simulink model "mrefrobotarm_modified_previous_y_previous_u_previous_ref"  (R2018b)
settings: Solver=FixedStepAuto  StartTime=0.0  StopTime=10  RelTol=1e-3  AbsTol=1e-6
undefined symbols (not defined in the file or in its folder): options, sfunxy2
libraries: neural x949, simulink x1
(part 15 of 31)

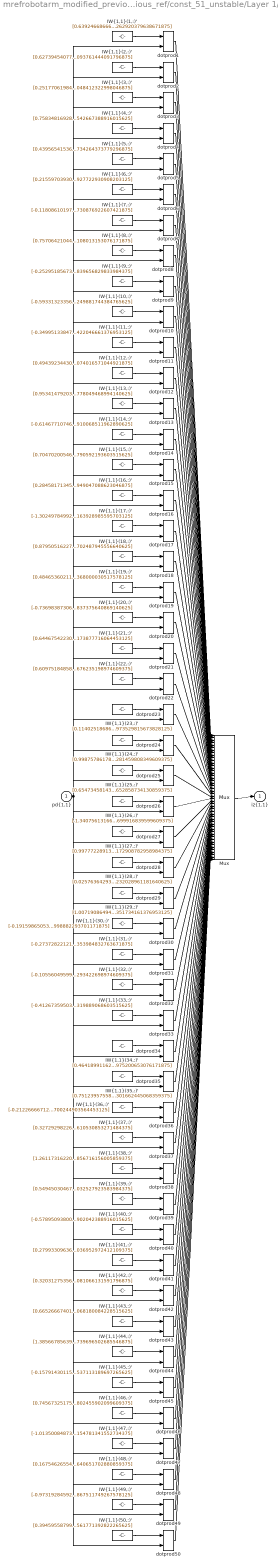
== system mrefrobotarm_modified_previous_y_previous_u_previous_ref/const_51_unstable/Layer 1/IW{1,1} ==
  "pd{1,1}" : Inport  PortDimensions=10
      mask Display: e = 0.06;c1 = [120 230 180]/255;c2 = ([120 230 180]+0)/(256+128);c3 = ([120 230 180]+128)/(256+128);patch([0 1 1 0],[0 0 1 1],c1);patch([0 1 1 1-e 1-e 0+e],[0 0 1 1-e 0+e 0+e],c2);patch([0 0 1 1-e 0+e 0+e],[0 1 1 1-e 1-e 0+e],c3);plot([0 1 1 0 0],[0 0 1 1 0]);
  "IW{1,1}(1,:)'" : Constant  Value=[0.63924668666616246692768754655844531953334808349609375;0.6942047904100672184313225443474948406219482421875;0.62567328865484228561655299927224405109882354736328125;0.261371173254488609050127934096963144838809967041015625;-0.177662377791001635518597367990878410637378692626953125;-0.8287859344063581712447330573922954499721527099609375;0.352973927789879848848642041048151440918445587158203125;0.2586532549009732395717264807899482548236846923828125;0.25408612949347031406688302013208158314228057861328125;-0.98861951008364001847183999416301958262920379638671875]
      mask Display: e = 0.06;c1 = [120 150 230]/255;c2 = ([120 150 230]+0)/383;c3 = ([120 150 230]+128)/383;patch([0 1 1 0],[0 0 1 1],c1);patch([0 1 1 1-e 1-e 0+e],[0 0 1 1-e 0+e 0+e],c2);patch([0 0 1 1-e 0+e 0+e],[0 1 1 1-e 1-e 0+e],c3);plot([0 1 1 0 0],[0 0 1 1 0]);disp('Weights');
  "IW{1,1}(10,:)'" : Constant  Value=[-0.59331323356992948792054676232510246336460113525390625;0.7977697325770243264031478247488848865032196044921875;-0.386101063294460644659267245515366084873676300048828125;-0.089448974061199615359640802125795744359493255615234375;0.50551080428874650696258186144405044615268707275390625;1.28460159328148382229528579046018421649932861328125;-1.051667369853578559713014328735880553722381591796875;-0.3071981244127155452616761976969428360462188720703125;-0.145228187797881769238728111304226331412792205810546875;0.416816636720638789004311774988309480249881744384765625]
      mask Display: e = 0.06;c1 = [120 150 230]/255;c2 = ([120 150 230]+0)/383;c3 = ([120 150 230]+128)/383;patch([0 1 1 0],[0 0 1 1],c1);patch([0 1 1 1-e 1-e 0+e],[0 0 1 1-e 0+e 0+e],c2);patch([0 0 1 1-e 0+e 0+e],[0 1 1 1-e 1-e 0+e],c3);plot([0 1 1 0 0],[0 0 1 1 0]);disp('Weights');
  "IW{1,1}(11,:)'" : Constant  Value=[-0.3499513384700432272467196526122279465198516845703125;-0.8005402749156467212543475397978909313678741455078125;-0.406764093260752357394949285662733018398284912109375;0.376972184217993555588321896721026860177516937255859375;-0.55931023341791130665257014697999693453311920166015625;-0.263639868612703442973810297189629636704921722412109375;-0.8852424690401410334317233719048090279102325439453125;0.51134822194627427283109000200056470930576324462890625;0.81875181176692046758347487411811016499996185302734375;0.45777739158591945756171526227262802422046661376953125]
      mask Display: e = 0.06;c1 = [120 150 230]/255;c2 = ([120 150 230]+0)/383;c3 = ([120 150 230]+128)/383;patch([0 1 1 0],[0 0 1 1],c1);patch([0 1 1 1-e 1-e 0+e],[0 0 1 1-e 0+e 0+e],c2);patch([0 0 1 1-e 0+e 0+e],[0 1 1 1-e 1-e 0+e],c3);plot([0 1 1 0 0],[0 0 1 1 0]);disp('Weights');
  "IW{1,1}(12,:)'" : Constant  Value=[0.494392344304093567242119888760498724877834320068359375;-1.09077574447859060313703594147227704524993896484375;-0.266408320699227540995224217112991027534008026123046875;-0.65079124667000576298647729345248080790042877197265625;-0.443937679832130116519550711018382571637630462646484375;0.334628474247073259828511027080821804702281951904296875;-0.7130336086197643918893618319998495280742645263671875;-1.161922006909116067419063256238587200641632080078125;-0.7882646426815498319484731837292201817035675048828125;-0.2961987538115529172699780247057788074016571044921875]
      mask Display: e = 0.06;c1 = [120 150 230]/255;c2 = ([120 150 230]+0)/383;c3 = ([120 150 230]+128)/383;patch([0 1 1 0],[0 0 1 1],c1);patch([0 1 1 1-e 1-e 0+e],[0 0 1 1-e 0+e 0+e],c2);patch([0 0 1 1-e 0+e 0+e],[0 1 1 1-e 1-e 0+e],c3);plot([0 1 1 0 0],[0 0 1 1 0]);disp('Weights');
  "IW{1,1}(13,:)'" : Constant  Value=[0.95341479203810586273704075210844166576862335205078125;-0.8400060597329204181704653819906525313854217529296875;-0.7955112231704415393096496700309216976165771484375;0.9668516464493592810214295241166837513446807861328125;-0.59452250697652286870464877210906706750392913818359375;-0.8387872006048218143092753962264396250247955322265625;0.15730537243195630292547093631583265960216522216796875;0.01305569298102214094436934743725942098535597324371337890625;-0.0997248402186528271062826433990267105400562286376953125;-0.048607066451850290678127208821024396456778049468994140625]
      mask Display: e = 0.06;c1 = [120 150 230]/255;c2 = ([120 150 230]+0)/383;c3 = ([120 150 230]+128)/383;patch([0 1 1 0],[0 0 1 1],c1);patch([0 1 1 1-e 1-e 0+e],[0 0 1 1-e 0+e 0+e],c2);patch([0 0 1 1-e 0+e 0+e],[0 1 1 1-e 1-e 0+e],c3);plot([0 1 1 0 0],[0 0 1 1 0]);disp('Weights');
  "IW{1,1}(14,:)'" : Constant  Value=[-0.61467710746125892029567694407887756824493408203125;-0.74682779167762614047632041547331027686595916748046875;-0.473858474488004943747654351682285778224468231201171875;-0.95402929876217867910526138075510971248149871826171875;0.333174273926396036227259855877491645514965057373046875;-0.36303307199912338010250323350192047655582427978515625;0.81652223062918627416451045064604841172695159912109375;0.2424313956082983778639317051784018985927104949951171875;-0.79565150315721100415800037808367051184177398681640625;-0.5094853025869279239401521408581174910068511962890625]
      mask Display: e = 0.06;c1 = [120 150 230]/255;c2 = ([120 150 230]+0)/383;c3 = ([120 150 230]+128)/383;patch([0 1 1 0],[0 0 1 1],c1);patch([0 1 1 1-e 1-e 0+e],[0 0 1 1-e 0+e 0+e],c2);patch([0 0 1 1-e 0+e 0+e],[0 1 1 1-e 1-e 0+e],c3);plot([0 1 1 0 0],[0 0 1 1 0]);disp('Weights');
  "IW{1,1}(15,:)'" : Constant  Value=[0.70470200546815409126111262594349682331085205078125;0.9721504333185293500463330929051153361797332763671875;0.626300057389828079834614982246421277523040771484375;0.213189582099907293244456241154693998396396636962890625;0.6913359965783083538326536654494702816009521484375;-0.00295197046113919621401766590906845522113144397735595703125;-0.8625857589857603979766054180799983441829681396484375;0.59018061405102095751118440603022463619709014892578125;0.90924827447133338420570680682430975139141082763671875;0.85333254725311835642287405789829790592193603515625]
      mask Display: e = 0.06;c1 = [120 150 230]/255;c2 = ([120 150 230]+0)/383;c3 = ([120 150 230]+128)/383;patch([0 1 1 0],[0 0 1 1],c1);patch([0 1 1 1-e 1-e 0+e],[0 0 1 1-e 0+e 0+e],c2);patch([0 0 1 1-e 0+e 0+e],[0 1 1 1-e 1-e 0+e],c3);plot([0 1 1 0 0],[0 0 1 1 0]);disp('Weights');
  "IW{1,1}(16,:)'" : Constant  Value=[0.284581713458217089307566993738873861730098724365234375;-0.280621549126129188334033415230805985629558563232421875;-1.03564915596999451707915795850567519664764404296875;-0.07172317120460820760730058509579976089298725128173828125;0.39460759001793388467405065966886468231678009033203125;0.9190004709601919952177695449790917336940765380859375;0.75048181864749563541039378833374939858913421630859375;0.81573633636398434898495679590268991887569427490234375;-0.03591301039200699152242890477282344363629817962646484375;0.85062050036111880313427491273614577949047088623046875]
      mask Display: e = 0.06;c1 = [120 150 230]/255;c2 = ([120 150 230]+0)/383;c3 = ([120 150 230]+128)/383;patch([0 1 1 0],[0 0 1 1],c1);patch([0 1 1 1-e 1-e 0+e],[0 0 1 1-e 0+e 0+e],c2);patch([0 0 1 1-e 0+e 0+e],[0 1 1 1-e 1-e 0+e],c3);plot([0 1 1 0 0],[0 0 1 1 0]);disp('Weights');
  "IW{1,1}(17,:)'" : Constant  Value=[-1.3024978499248760499540367163717746734619140625;1.3419509605779460503782729574595578014850616455078125;-0.504540389310853765181263952399604022502899169921875;0.5007126364069047763649678017827682197093963623046875;-0.2241232702447646107923873159961658529937267303466796875;-0.682842349014617155944506521336734294891357421875;-0.59445267552896596807698870179592631757259368896484375;1.2325888373718640877996222116053104400634765625;-0.0831161952569162976178773760693729855120182037353515625;-0.565871713313782720433664508163928985595703125]
      mask Display: e = 0.06;c1 = [120 150 230]/255;c2 = ([120 150 230]+0)/383;c3 = ([120 150 230]+128)/383;patch([0 1 1 0],[0 0 1 1],c1);patch([0 1 1 1-e 1-e 0+e],[0 0 1 1-e 0+e 0+e],c2);patch([0 0 1 1-e 0+e 0+e],[0 1 1 1-e 1-e 0+e],c3);plot([0 1 1 0 0],[0 0 1 1 0]);disp('Weights');
  "IW{1,1}(18,:)'" : Constant  Value=[0.87950516227352704135000749374739825725555419921875;-1.1836890447335763898450977649190463125705718994140625;0.530743319631852283890793842147104442119598388671875;0.25272269822145509987620926040108315646648406982421875;0.3653029490932790945834085505339317023754119873046875;-0.3810355298209933128106285948888398706912994384765625;-0.64649896901114478620087311355746351182460784912109375;0.300211636084151523018448415314196608960628509521484375;-0.428387989166555904763100670606945641338825225830078125;0.1751370188022575435926597720026620663702487945556640625]
      mask Display: e = 0.06;c1 = [120 150 230]/255;c2 = ([120 150 230]+0)/383;c3 = ([120 150 230]+128)/383;patch([0 1 1 0],[0 0 1 1],c1);patch([0 1 1 1-e 1-e 0+e],[0 0 1 1-e 0+e 0+e],c2);patch([0 0 1 1-e 0+e 0+e],[0 1 1 1-e 1-e 0+e],c3);plot([0 1 1 0 0],[0 0 1 1 0]);disp('Weights');
  "IW{1,1}(19,:)'" : Constant  Value=[0.48465360211071384366476877403329126536846160888671875;-0.71564584780320006363041329677798785269260406494140625;-0.1134074702547006319175437738522305153310298919677734375;-0.38993116043481312882335032554692588746547698974609375;-0.6878127659446697794720648744259960949420928955078125;0.364118141393751260093125665662228129804134368896484375;0.472555272999996500704611435139668174088001251220703125;0.1810251256197520641766374183134757913649082183837890625;-0.86523040981986676367654354180558584630489349365234375;0.479601809228045461441780616951291449368000030517578125]
      mask Display: e = 0.06;c1 = [120 150 230]/255;c2 = ([120 150 230]+0)/383;c3 = ([120 150 230]+128)/383;patch([0 1 1 0],[0 0 1 1],c1);patch([0 1 1 1-e 1-e 0+e],[0 0 1 1-e 0+e 0+e],c2);patch([0 0 1 1-e 0+e 0+e],[0 1 1 1-e 1-e 0+e],c3);plot([0 1 1 0 0],[0 0 1 1 0]);disp('Weights');
  "IW{1,1}(2,:)'" : Constant  Value=[0.62739454077566769729656925846938975155353546142578125;0.76646187434358548085100437674554996192455291748046875;0.8709533037536247856991167282103560864925384521484375;-0.7335425158669657275112285788054578006267547607421875;-0.2353430122977316074628362230214406736195087432861328125;0.81640575167049933558161001201369799673557281494140625;0.72409700386967756902123483087052591145038604736328125;0.45266443098558573066014787400490604341030120849609375;0.1720296099524863675522823314167908392846584320068359375;-1.033946502245487675253343695658259093761444091796875]
      mask Display: e = 0.06;c1 = [120 150 230]/255;c2 = ([120 150 230]+0)/383;c3 = ([120 150 230]+128)/383;patch([0 1 1 0],[0 0 1 1],c1);patch([0 1 1 1-e 1-e 0+e],[0 0 1 1-e 0+e 0+e],c2);patch([0 0 1 1-e 0+e 0+e],[0 1 1 1-e 1-e 0+e],c3);plot([0 1 1 0 0],[0 0 1 1 0]);disp('Weights');
  "IW{1,1}(20,:)'" : Constant  Value=[-0.7369838730691868899924656943767331540584564208984375;-0.45128021209423885284905963999335654079914093017578125;0.84230940906155671310528987305588088929653167724609375;-0.13210537730959004409925228173960931599140167236328125;-0.0816075728062311822608165812198421917855739593505859375;-0.022981247943674322498086581845200271345674991607666015625;-0.41000811331266484582869225050671957433223724365234375;-0.77313035067709401371160993221565149724483489990234375;1.1472657437635669364084378685220144689083099365234375;0.65177088639075508869069608408608473837375640869140625]
      mask Display: e = 0.06;c1 = [120 150 230]/255;c2 = ([120 150 230]+0)/383;c3 = ([120 150 230]+128)/383;patch([0 1 1 0],[0 0 1 1],c1);patch([0 1 1 1-e 1-e 0+e],[0 0 1 1-e 0+e 0+e],c2);patch([0 0 1 1-e 0+e 0+e],[0 1 1 1-e 1-e 0+e],c3);plot([0 1 1 0 0],[0 0 1 1 0]);disp('Weights');
  "IW{1,1}(21,:)'" : Constant  Value=[0.64467542230901309086021910843555815517902374267578125;-0.365686964333162556339829052376444451510906219482421875;-1.1167429230065206713362613299977965652942657470703125;-0.28027872976577128394382043552468530833721160888671875;-1.15425342475938119690681560314260423183441162109375;0.00147963811568855956035672960524607333354651927947998046875;-0.58953701284011483796376751342904753983020782470703125;-0.8196672851852664365424061543308198451995849609375;0.5859115741298446256024590184097178280353546142578125;-0.232936107706306405606966336563345976173877716064453125]
      mask Display: e = 0.06;c1 = [120 150 230]/255;c2 = ([120 150 230]+0)/383;c3 = ([120 150 230]+128)/383;patch([0 1 1 0],[0 0 1 1],c1);patch([0 1 1 1-e 1-e 0+e],[0 0 1 1-e 0+e 0+e],c2);patch([0 0 1 1-e 0+e 0+e],[0 1 1 1-e 1-e 0+e],c3);plot([0 1 1 0 0],[0 0 1 1 0]);disp('Weights');
  "IW{1,1}(22,:)'" : Constant  Value=[0.60975184858876441129638124039047397673130035400390625;-1.1137511038478298264209342960384674370288848876953125;0.75737428038547705000382848083972930908203125;-0.949374181419179397067864556447602808475494384765625;-0.05697986041225151787603664388370816595852375030517578125;-0.232736767374490505222439651333843357861042022705078125;-0.306641934219895606617001249105669558048248291015625;0.5422382160818004503965994445024989545345306396484375;0.355223820942887125173825779711478389799594879150390625;0.520671647549169502866561742848716676235198974609375]
      mask Display: e = 0.06;c1 = [120 150 230]/255;c2 = ([120 150 230]+0)/383;c3 = ([120 150 230]+128)/383;patch([0 1 1 0],[0 0 1 1],c1);patch([0 1 1 1-e 1-e 0+e],[0 0 1 1-e 0+e 0+e],c2);patch([0 0 1 1-e 0+e 0+e],[0 1 1 1-e 1-e 0+e],c3);plot([0 1 1 0 0],[0 0 1 1 0]);disp('Weights');
  "IW{1,1}(23,:)'" : Constant  Value=[0.11402518686013463078410268281004391610622406005859375;0.4904421195008132894344043961609713733196258544921875;0.68664774896037561457973197320825420320034027099609375;0.51860306312847981313751688503543846309185028076171875;-0.6427156453918172474004677496850490570068359375;-0.9590374190953838695605782049824483692646026611328125;0.0373927440447821834990094203021726571023464202880859375;0.68495669364243438881345582558424212038516998291015625;0.94546553725292736825025485813966952264308929443359375;-0.339602270344673329294238328657229430973529815673828125]
      mask Display: e = 0.06;c1 = [120 150 230]/255;c2 = ([120 150 230]+0)/383;c3 = ([120 150 230]+128)/383;patch([0 1 1 0],[0 0 1 1],c1);patch([0 1 1 1-e 1-e 0+e],[0 0 1 1-e 0+e 0+e],c2);patch([0 0 1 1-e 0+e 0+e],[0 1 1 1-e 1-e 0+e],c3);plot([0 1 1 0 0],[0 0 1 1 0]);disp('Weights');
  "IW{1,1}(24,:)'" : Constant  Value=[0.9987578617813903658628760240389965474605560302734375;0.495486441201053506855345176518312655389308929443359375;-0.2127739742921361532079771450298721902072429656982421875;0.8271982061539644437431206824840046465396881103515625;-0.410956095251641340126980139757506549358367919921875;-0.7970129128845797605862344425986520946025848388671875;0.9105423389600943995247916973312385380268096923828125;0.90778107591924384056625285666086710989475250244140625;-0.506466458102025729459683134336955845355987548828125;0.354856883470640871447443487340933643281459808349609375]
      mask Display: e = 0.06;c1 = [120 150 230]/255;c2 = ([120 150 230]+0)/383;c3 = ([120 150 230]+128)/383;patch([0 1 1 0],[0 0 1 1],c1);patch([0 1 1 1-e 1-e 0+e],[0 0 1 1-e 0+e 0+e],c2);patch([0 0 1 1-e 0+e 0+e],[0 1 1 1-e 1-e 0+e],c3);plot([0 1 1 0 0],[0 0 1 1 0]);disp('Weights');
  "IW{1,1}(25,:)'" : Constant  Value=[0.6547345814357929949522940660244785249233245849609375;0.39845260412756022816438417066819965839385986328125;-0.1830170343104607078021928145972196944057941436767578125;1.3632995620440577777543467163923196494579315185546875;0.80754118590340340233524329960346221923828125;0.381451563537807292192383101792074739933013916015625;0.71053106300381696502910244817030616104602813720703125;-0.63610894017396069077818765435949899256229400634765625;0.363044771167251700827449667485780082643032073974609375;-0.042781005916550096657147150835953652858734130859375]
      mask Display: e = 0.06;c1 = [120 150 230]/255;c2 = ([120 150 230]+0)/383;c3 = ([120 150 230]+128)/383;patch([0 1 1 0],[0 0 1 1],c1);patch([0 1 1 1-e 1-e 0+e],[0 0 1 1-e 0+e 0+e],c2);patch([0 0 1 1-e 0+e 0+e],[0 1 1 1-e 1-e 0+e],c3);plot([0 1 1 0 0],[0 0 1 1 0]);disp('Weights');
  "IW{1,1}(26,:)'" : Constant  Value=[-1.340756131664672334835586298140697181224822998046875;0.27007456478198499372211927038733847439289093017578125;-0.039195464485621826777883569548066589049994945526123046875;-0.62996699208041062600926807135692797601222991943359375;1.24456451050825744886196844163350760936737060546875;-0.25402186930486736482492915456532500684261322021484375;0.29241835179487962736999406843096949160099029541015625;-0.2364904402252494819425265859536011703312397003173828125;-0.56760479989431023017942834485438652336597442626953125;0.419969212660492308142323736319667659699916839599609375]
      mask Display: e = 0.06;c1 = [120 150 230]/255;c2 = ([120 150 230]+0)/383;c3 = ([120 150 230]+128)/383;patch([0 1 1 0],[0 0 1 1],c1);patch([0 1 1 1-e 1-e 0+e],[0 0 1 1-e 0+e 0+e],c2);patch([0 0 1 1-e 0+e 0+e],[0 1 1 1-e 1-e 0+e],c3);plot([0 1 1 0 0],[0 0 1 1 0]);disp('Weights');
  "IW{1,1}(27,:)'" : Constant  Value=[0.9977722891376490377268737574922852218151092529296875;-0.6068679135028485216452054373803548514842987060546875;0.50421216035368698893393002435914240777492523193359375;0.311630050128098357031802834171685390174388885498046875;-0.37280063608242486328236964254756458103656768798828125;0.97080864432455837853552793603739701211452484130859375;-1.060044686277588521505776952835731208324432373046875;0.97769244225342089027463998718303628265857696533203125;-0.329571569628752059077925196106662042438983917236328125;-0.456574952393950128648469899417250417172908782958984375]
      mask Display: e = 0.06;c1 = [120 150 230]/255;c2 = ([120 150 230]+0)/383;c3 = ([120 150 230]+128)/383;patch([0 1 1 0],[0 0 1 1],c1);patch([0 1 1 1-e 1-e 0+e],[0 0 1 1-e 0+e 0+e],c2);patch([0 0 1 1-e 0+e 0+e],[0 1 1 1-e 1-e 0+e],c3);plot([0 1 1 0 0],[0 0 1 1 0]);disp('Weights');
  "IW{1,1}(28,:)'" : Constant  Value=[0.02576364293666101590307704327642568387091159820556640625;-0.65255059643876556219055373730952851474285125732421875;-0.87832867100243394720138212505844421684741973876953125;-0.778813682076582747271231710328720510005950927734375;-0.709411760323691797935907743521966040134429931640625;0.5312754913211226170943746183183975517749786376953125;0.501196663942328424212746540433727204799652099609375;-0.6671465678213934769047455120016820728778839111328125;-0.56260016957891745281727935434901155531406402587890625;-0.56810980620226703141639745808788575232028961181640625]
      mask Display: e = 0.06;c1 = [120 150 230]/255;c2 = ([120 150 230]+0)/383;c3 = ([120 150 230]+128)/383;patch([0 1 1 0],[0 0 1 1],c1);patch([0 1 1 1-e 1-e 0+e],[0 0 1 1-e 0+e 0+e],c2);patch([0 0 1 1-e 0+e 0+e],[0 1 1 1-e 1-e 0+e],c3);plot([0 1 1 0 0],[0 0 1 1 0]);disp('Weights');
  "IW{1,1}(29,:)'" : Constant  Value=[1.0071908649480600939085661593708209693431854248046875;-0.59269777759990216470242785362643189728260040283203125;0.6430474184332164444555246518575586378574371337890625;-0.177195096398686136041078498237766325473785400390625;0.64647725132764144451158472293172962963581085205078125;-1.0737955968979908671911971396184526383876800537109375;0.32481199487106326984076076769270002841949462890625;0.2653582624213639551413734807283617556095123291015625;0.32551897435131615932135673574521206319332122802734375;0.421670984283849581419900687251356430351734161376953125]
      mask Display: e = 0.06;c1 = [120 150 230]/255;c2 = ([120 150 230]+0)/383;c3 = ([120 150 230]+128)/383;patch([0 1 1 0],[0 0 1 1],c1);patch([0 1 1 1-e 1-e 0+e],[0 0 1 1-e 0+e 0+e],c2);patch([0 0 1 1-e 0+e 0+e],[0 1 1 1-e 1-e 0+e],c3);plot([0 1 1 0 0],[0 0 1 1 0]);disp('Weights');
  "IW{1,1}(3,:)'" : Constant  Value=[0.251770619842439924429555730966967530548572540283203125;-0.29186179488348640287398438886157236993312835693359375;0.2317864436403720418411467107944190502166748046875;0.346406667185564176580925277448841370642185211181640625;-1.1818576323231848590467052417807281017303466796875;0.6938375834008052578383285435847938060760498046875;-0.95315078904075634103065794988651759922504425048828125;0.036065412262522460185021344614142435602843761444091796875;-0.6930875611524214274794530865619890391826629638671875;-0.72257924625952252295491007316741161048412322998046875]
      mask Display: e = 0.06;c1 = [120 150 230]/255;c2 = ([120 150 230]+0)/383;c3 = ([120 150 230]+128)/383;patch([0 1 1 0],[0 0 1 1],c1);patch([0 1 1 1-e 1-e 0+e],[0 0 1 1-e 0+e 0+e],c2);patch([0 0 1 1-e 0+e 0+e],[0 1 1 1-e 1-e 0+e],c3);plot([0 1 1 0 0],[0 0 1 1 0]);disp('Weights');
  "IW{1,1}(30,:)'" : Constant  Value=[-0.19159865053693125869216373757808469235897064208984375;-1.044827388502894915944807507912628352642059326171875;-0.95362540357193303908189818685059435665607452392578125;0.9439417571944748175383210764266550540924072265625;-0.776251292475051979380396005581133067607879638671875;0.062431350981061985161435501368032419122755527496337890625;-0.07510985747671532208880051939559052698314189910888671875;0.2325848996406161550698499240752425976097583770751953125;-0.441251057412189340301011952760745771229267120361328125;-0.1266650210668011922177100814224104396998882293701171875]
      mask Display: e = 0.06;c1 = [120 150 230]/255;c2 = ([120 150 230]+0)/383;c3 = ([120 150 230]+128)/383;patch([0 1 1 0],[0 0 1 1],c1);patch([0 1 1 1-e 1-e 0+e],[0 0 1 1-e 0+e 0+e],c2);patch([0 0 1 1-e 0+e 0+e],[0 1 1 1-e 1-e 0+e],c3);plot([0 1 1 0 0],[0 0 1 1 0]);disp('Weights');
  "IW{1,1}(31,:)'" : Constant  Value=[-0.27372822121770479242286455701105296611785888671875;-0.216348771194250166782779842833406291902065277099609375;-0.72304138575442433722884061353397555649280548095703125;-0.64024653526934127700798171645146794617176055908203125;-0.54564834135397799474986868517589755356311798095703125;1.00143652126254867340549026266671717166900634765625;-0.65234906555163518770967812088201753795146942138671875;-0.69565204535261149221270216003176756203174591064453125;-0.422829370206151355926493806691723875701427459716796875;0.79132190290408288557699734155903570353984832763671875]
      mask Display: e = 0.06;c1 = [120 150 230]/255;c2 = ([120 150 230]+0)/383;c3 = ([120 150 230]+128)/383;patch([0 1 1 0],[0 0 1 1],c1);patch([0 1 1 1-e 1-e 0+e],[0 0 1 1-e 0+e 0+e],c2);patch([0 0 1 1-e 0+e 0+e],[0 1 1 1-e 1-e 0+e],c3);plot([0 1 1 0 0],[0 0 1 1 0]);disp('Weights');
  "IW{1,1}(32,:)'" : Constant  Value=[-0.10556049599311063957873813023979892022907733917236328125;0.00584291461163955437585482144413617788814008235931396484375;-1.3863775039244092823764731292612850666046142578125;-0.2103211703886511685368532198481261730194091796875;-1.2577814118814940602675278569222427904605865478515625;0.05686350527750520800207567617690074257552623748779296875;0.40230834706792129029651050586835481226444244384765625;0.345830932655557699018089579112711362540721893310546875;-0.058080826938076889065509789134011953137814998626708984375;-0.78958512148689441456639315219945274293422698974609375]
      mask Display: e = 0.06;c1 = [120 150 230]/255;c2 = ([120 150 230]+0)/383;c3 = ([120 150 230]+128)/383;patch([0 1 1 0],[0 0 1 1],c1);patch([0 1 1 1-e 1-e 0+e],[0 0 1 1-e 0+e 0+e],c2);patch([0 0 1 1-e 0+e 0+e],[0 1 1 1-e 1-e 0+e],c3);plot([0 1 1 0 0],[0 0 1 1 0]);disp('Weights');
  "IW{1,1}(33,:)'" : Constant  Value=[-0.412673595033445028690266553894616663455963134765625;-0.61251027096036037011828057075035758316516876220703125;0.31789585632212757904113686890923418104648590087890625;0.49313760996205580067197615790064446628093719482421875;-0.76689035985725428901105260592885315418243408203125;0.92766504905938484970562285525375045835971832275390625;-0.81904960000742443870791476001613773405551910400390625;0.418870210355308192351486695770290680229663848876953125;0.0958785722800684914179925044663832522928714752197265625;0.393281295541891451339466811987222172319889068603515625]
      mask Display: e = 0.06;c1 = [120 150 230]/255;c2 = ([120 150 230]+0)/383;c3 = ([120 150 230]+128)/383;patch([0 1 1 0],[0 0 1 1],c1);patch([0 1 1 1-e 1-e 0+e],[0 0 1 1-e 0+e 0+e],c2);patch([0 0 1 1-e 0+e 0+e],[0 1 1 1-e 1-e 0+e],c3);plot([0 1 1 0 0],[0 0 1 1 0]);disp('Weights');
  "IW{1,1}(34,:)'" : Constant  Value=[0.4641899116284331494597381606581620872020721435546875;1.058282155187232564941268719849176704883575439453125;-0.302014535432015396310134747182019054889678955078125;-0.6903925305826994485158820680226199328899383544921875;0.61960402696297156577287523759878240525722503662109375;0.82478305479356517349032174024614505469799041748046875;-0.57352396235207991903592983362614177167415618896484375;0.1844165746886447243557682895698235370218753814697265625;1.063607222221527148775521709467284381389617919921875;0.030075523509437478153483169762694160453975200653076171875]
      mask Display: e = 0.06;c1 = [120 150 230]/255;c2 = ([120 150 230]+0)/383;c3 = ([120 150 230]+128)/383;patch([0 1 1 0],[0 0 1 1],c1);patch([0 1 1 1-e 1-e 0+e],[0 0 1 1-e 0+e 0+e],c2);patch([0 0 1 1-e 0+e 0+e],[0 1 1 1-e 1-e 0+e],c3);plot([0 1 1 0 0],[0 0 1 1 0]);disp('Weights');
  "IW{1,1}(35,:)'" : Constant  Value=[0.75123957558842124893061509283143095672130584716796875;-0.7965275034147210053703247467637993395328521728515625;0.045205342260291096756485984542450751177966594696044921875;-0.5146427157032678056935992572107352316379547119140625;-1.170604211533416094681570029933936893939971923828125;1.1039268224372966731294809505925513803958892822265625;-0.437798827711881555213579986229888163506984710693359375;0.336384367120219851532425536788650788366794586181640625;0.1421463715218020673614063298373366706073284149169921875;0.73457620854121896680766212739399634301662445068359375]
      mask Display: e = 0.06;c1 = [120 150 230]/255;c2 = ([120 150 230]+0)/383;c3 = ([120 150 230]+128)/383;patch([0 1 1 0],[0 0 1 1],c1);patch([0 1 1 1-e 1-e 0+e],[0 0 1 1-e 0+e 0+e],c2);patch([0 0 1 1-e 0+e 0+e],[0 1 1 1-e 1-e 0+e],c3);plot([0 1 1 0 0],[0 0 1 1 0]);disp('Weights');
  "IW{1,1}(36,:)'" : Constant  Value=[-0.2122666671298679974544398874058970250189304351806640625;0.76651151168379116906947956522344611585140228271484375;-0.0003967882681511071367441711998935716110281646251678466796875;0.44828287097590535648095055876183323562145233154296875;-0.5292928794968714267810128148994408547878265380859375;-0.8290689229590098019428978659561835229396820068359375;0.348926523801390942036704245765577070415019989013671875;1.014816697147457258409986025071702897548675537109375;-1.11439146435958935654753076960332691669464111328125;0.314956379104058659113007934138295240700244903564453125]
      mask Display: e = 0.06;c1 = [120 150 230]/255;c2 = ([120 150 230]+0)/383;c3 = ([120 150 230]+128)/383;patch([0 1 1 0],[0 0 1 1],c1);patch([0 1 1 1-e 1-e 0+e],[0 0 1 1-e 0+e 0+e],c2);patch([0 0 1 1-e 0+e 0+e],[0 1 1 1-e 1-e 0+e],c3);plot([0 1 1 0 0],[0 0 1 1 0]);disp('Weights');
  "IW{1,1}(37,:)'" : Constant  Value=[0.327292982263773513107452117765205912292003631591796875;0.8200236668707205911488244964857585728168487548828125;-0.201589082457516166613231689552776515483856201171875;0.37970567032044943989177454568562097847461700439453125;-0.61236992485544139430686527703073807060718536376953125;0.6132460084698820867998847461421974003314971923828125;-0.054611185509608493882094393256920739077031612396240234375;0.1957005208180704614040479327741195447742938995361328125;1.1601839643593023776446671035955660045146942138671875;-0.66306043780564338785410427590250037610530853271484375]
      mask Display: e = 0.06;c1 = [120 150 230]/255;c2 = ([120 150 230]+0)/383;c3 = ([120 150 230]+128)/383;patch([0 1 1 0],[0 0 1 1],c1);patch([0 1 1 1-e 1-e 0+e],[0 0 1 1-e 0+e 0+e],c2);patch([0 0 1 1-e 0+e 0+e],[0 1 1 1-e 1-e 0+e],c3);plot([0 1 1 0 0],[0 0 1 1 0]);disp('Weights');
  "IW{1,1}(38,:)'" : Constant  Value=[1.2611731622048385492718125533428974449634552001953125;0.75217689002794940744678342525730840861797332763671875;-0.44177672716117732942819884556229226291179656982421875;0.1614755608187066482361871067041647620499134063720703125;0.56127082889771517937305134182679466903209686279296875;0.06362120657116472621783742624756996519863605499267578125;-0.395335106460912577563959757753764279186725616455078125;0.256862891181286523423210610417299903929233551025390625;0.3661751044816645705992641524062491953372955322265625;1.056856092282413950300679061911068856716156005859375]
      mask Display: e = 0.06;c1 = [120 150 230]/255;c2 = ([120 150 230]+0)/383;c3 = ([120 150 230]+128)/383;patch([0 1 1 0],[0 0 1 1],c1);patch([0 1 1 1-e 1-e 0+e],[0 0 1 1-e 0+e 0+e],c2);patch([0 0 1 1-e 0+e 0+e],[0 1 1 1-e 1-e 0+e],c3);plot([0 1 1 0 0],[0 0 1 1 0]);disp('Weights');
  "IW{1,1}(39,:)'" : Constant  Value=[0.54945030467812527863458171850652433931827545166015625;0.703318019555827067534892194089479744434356689453125;-0.47129170864535330220945752444094978272914886474609375;-0.66171117079673946737017331543029285967350006103515625;-0.3313444525024393794154775605420581996440887451171875;-1.0659555616150149237597588580683805048465728759765625;-0.1805959793510603927924051959053031168878078460693359375;0.12402759728644989489776406799137475900352001190185546875;1.18785882888554450431684017530642449855804443359375;0.2004042787787728430171085847177891992032527923583984375]
      mask Display: e = 0.06;c1 = [120 150 230]/255;c2 = ([120 150 230]+0)/383;c3 = ([120 150 230]+128)/383;patch([0 1 1 0],[0 0 1 1],c1);patch([0 1 1 1-e 1-e 0+e],[0 0 1 1-e 0+e 0+e],c2);patch([0 0 1 1-e 0+e 0+e],[0 1 1 1-e 1-e 0+e],c3);plot([0 1 1 0 0],[0 0 1 1 0]);disp('Weights');
  "IW{1,1}(4,:)'" : Constant  Value=[0.75834816928748216557920613922760821878910064697265625;-0.425134316807037226926269113391754217445850372314453125;0.789199870866053476703427804750390350818634033203125;-0.483839144032371659687186138398828916251659393310546875;-0.035315395379454724011925037530090776272118091583251953125;-1.0588470574337256469021895100013352930545806884765625;-0.64788678209714711808686615768237970769405364990234375;0.024723409091161600847907919842327828519046306610107421875;0.91343338461698364572072250666678883135318756103515625;-0.177623441896880562840266293278546072542667388916015625]
      mask Display: e = 0.06;c1 = [120 150 230]/255;c2 = ([120 150 230]+0)/383;c3 = ([120 150 230]+128)/383;patch([0 1 1 0],[0 0 1 1],c1);patch([0 1 1 1-e 1-e 0+e],[0 0 1 1-e 0+e 0+e],c2);patch([0 0 1 1-e 0+e 0+e],[0 1 1 1-e 1-e 0+e],c3);plot([0 1 1 0 0],[0 0 1 1 0]);disp('Weights');
  "IW{1,1}(40,:)'" : Constant  Value=[-0.57895093800558183882998264380148611962795257568359375;0.1843102464098818338289476059799198992550373077392578125;0.46800026883722001258547606994397938251495361328125;1.0861561313280019280824717498035170137882232666015625;0.6081916099333486425138062259065918624401092529296875;0.0358858083335172606265217609688988886773586273193359375;-0.140409969834986603220983170103863812983036041259765625;0.986851124889954522956259097554720938205718994140625;0.24349297587613116800042689646943472325801849365234375;-0.78559549561909902681833273163647390902042388916015625]
      mask Display: e = 0.06;c1 = [120 150 230]/255;c2 = ([120 150 230]+0)/383;c3 = ([120 150 230]+128)/383;patch([0 1 1 0],[0 0 1 1],c1);patch([0 1 1 1-e 1-e 0+e],[0 0 1 1-e 0+e 0+e],c2);patch([0 0 1 1-e 0+e 0+e],[0 1 1 1-e 1-e 0+e],c3);plot([0 1 1 0 0],[0 0 1 1 0]);disp('Weights');
  "IW{1,1}(41,:)'" : Constant  Value=[0.27993309636441254806271672350703738629817962646484375;0.48871251903327361798545780402491800487041473388671875;-0.66773317165742651635440552126965485513210296630859375;0.5340539295473434311389837603201158344745635986328125;0.270886623086703026697108498410671018064022064208984375;1.18303452379921214543401219998486340045928955078125;-0.994656396841185230783821680233813822269439697265625;-0.90432543338826676393438219747622497379779815673828125;0.860977276785207745746220098226331174373626708984375;-0.40537272176258587474961814223206602036952972412109375]
      mask Display: e = 0.06;c1 = [120 150 230]/255;c2 = ([120 150 230]+0)/383;c3 = ([120 150 230]+128)/383;patch([0 1 1 0],[0 0 1 1],c1);patch([0 1 1 1-e 1-e 0+e],[0 0 1 1-e 0+e 0+e],c2);patch([0 0 1 1-e 0+e 0+e],[0 1 1 1-e 1-e 0+e],c3);plot([0 1 1 0 0],[0 0 1 1 0]);disp('Weights');
  "IW{1,1}(42,:)'" : Constant  Value=[0.320312753560126617369263612999930046498775482177734375;0.29911598860352917039762132844771258533000946044921875;0.76467042336051294082466256440966390073299407958984375;0.2429615673984670820573228411376476287841796875;0.214771692171215777822368409033515490591526031494140625;0.08608691671594137506673405368928797543048858642578125;1.2147349653145529391196077995118685066699981689453125;1.3191982752785935684158857839065603911876678466796875;0.6397056681883446227487866053706966340541839599609375;0.2243206762358684602798319929206627421081066131591796875]
      mask Display: e = 0.06;c1 = [120 150 230]/255;c2 = ([120 150 230]+0)/383;c3 = ([120 150 230]+128)/383;patch([0 1 1 0],[0 0 1 1],c1);patch([0 1 1 1-e 1-e 0+e],[0 0 1 1-e 0+e 0+e],c2);patch([0 0 1 1-e 0+e 0+e],[0 1 1 1-e 1-e 0+e],c3);plot([0 1 1 0 0],[0 0 1 1 0]);disp('Weights');
  "IW{1,1}(43,:)'" : Constant  Value=[0.66526667401786543365460602217353880405426025390625;-0.62196190985420407582040525085176341235637664794921875;0.9507469436317894651011783935246057808399200439453125;0.425021240222747509474032767684548161923885345458984375;-0.11362166042913411645454146992051391862332820892333984375;-0.79374103463417056136819383027614094316959381103515625;0.80072400276515864891990759133477695286273956298828125;-0.869784005513377422857956844381988048553466796875;0.9619517363130665188464263337664306163787841796875;-0.60540679655290985383686575005413033068180084228515625]
      mask Display: e = 0.06;c1 = [120 150 230]/255;c2 = ([120 150 230]+0)/383;c3 = ([120 150 230]+128)/383;patch([0 1 1 0],[0 0 1 1],c1);patch([0 1 1 1-e 1-e 0+e],[0 0 1 1-e 0+e 0+e],c2);patch([0 0 1 1-e 0+e 0+e],[0 1 1 1-e 1-e 0+e],c3);plot([0 1 1 0 0],[0 0 1 1 0]);disp('Weights');
  "IW{1,1}(44,:)'" : Constant  Value=[1.3856678563957169902920441018068231642246246337890625;0.480591477899259433836931521000224165618419647216796875;-0.50186481969417073845107779561658389866352081298828125;0.0637851739995955735462729307982954196631908416748046875;-0.95842067382357998273079147111275233328342437744140625;-0.9809686933629475635854078063857741653919219970703125;-0.33919887334723541894021536791115067899227142333984375;-0.052180742349234698895799056117539294064044952392578125;-0.0799843421390668829484837942800368182361125946044921875;0.36868331004489363067477825097739696502685546875]
      mask Display: e = 0.06;c1 = [120 150 230]/255;c2 = ([120 150 230]+0)/383;c3 = ([120 150 230]+128)/383;patch([0 1 1 0],[0 0 1 1],c1);patch([0 1 1 1-e 1-e 0+e],[0 0 1 1-e 0+e 0+e],c2);patch([0 0 1 1-e 0+e 0+e],[0 1 1 1-e 1-e 0+e],c3);plot([0 1 1 0 0],[0 0 1 1 0]);disp('Weights');
  "IW{1,1}(45,:)'" : Constant  Value=[-0.15791430115240545628552126800059340894222259521484375;0.52096310830967074156916396532324142754077911376953125;1.07312165486326716035136996651999652385711669921875;-0.00831058744162140559941231998664079583249986171722412109375;0.849527546798957811091668190783821046352386474609375;0.9407957737111407592323075732565484941005706787109375;-0.1623557661142418784283592003703233785927295684814453125;-1.03385069274804042294135797419585287570953369140625;-0.49595759084346402456588975837803445756435394287109375;-0.58309357977172260323328600861714221537113189697265625]
      mask Display: e = 0.06;c1 = [120 150 230]/255;c2 = ([120 150 230]+0)/383;c3 = ([120 150 230]+128)/383;patch([0 1 1 0],[0 0 1 1],c1);patch([0 1 1 1-e 1-e 0+e],[0 0 1 1-e 0+e 0+e],c2);patch([0 0 1 1-e 0+e 0+e],[0 1 1 1-e 1-e 0+e],c3);plot([0 1 1 0 0],[0 0 1 1 0]);disp('Weights');
  "IW{1,1}(46,:)'" : Constant  Value=[0.74567325175636900436160203753388486802577972412109375;-0.687527025083957799012068790034390985965728759765625;0.233184524485493593903839837366831488907337188720703125;-0.976664837800916618704150096164084970951080322265625;-0.1703463863294059355002474376306054182350635528564453125;1.1290308875096537466475865585380233824253082275390625;-0.004982561947859391604520595819849404506385326385498046875;-0.0308258315524873489910095969435133156366646289825439453125;0.9342374214499764573105267118080519139766693115234375;-0.2266618960853551134615457840482122264802455902099609375]
      mask Display: e = 0.06;c1 = [120 150 230]/255;c2 = ([120 150 230]+0)/383;c3 = ([120 150 230]+128)/383;patch([0 1 1 0],[0 0 1 1],c1);patch([0 1 1 1-e 1-e 0+e],[0 0 1 1-e 0+e 0+e],c2);patch([0 0 1 1-e 0+e 0+e],[0 1 1 1-e 1-e 0+e],c3);plot([0 1 1 0 0],[0 0 1 1 0]);disp('Weights');
  "IW{1,1}(47,:)'" : Constant  Value=[-1.0135008487368033502917796795372851192951202392578125;-0.402975437106179390500670933761284686625003814697265625;-0.726066246859837338689658281509764492511749267578125;0.0026805782390963016521834294536574816447682678699493408203125;0.1659127456605878070394766155004617758095264434814453125;0.6781263157839181321406840652343817055225372314453125;0.131450293805944085079318028874695301055908203125;1.317987506604807901311460227589122951030731201171875;-0.67583510105865840511540909574250690639019012451171875;0.0927649628941927539838019356466247700154781341552734375]
      mask Display: e = 0.06;c1 = [120 150 230]/255;c2 = ([120 150 230]+0)/383;c3 = ([120 150 230]+128)/383;patch([0 1 1 0],[0 0 1 1],c1);patch([0 1 1 1-e 1-e 0+e],[0 0 1 1-e 0+e 0+e],c2);patch([0 0 1 1-e 0+e 0+e],[0 1 1 1-e 1-e 0+e],c3);plot([0 1 1 0 0],[0 0 1 1 0]);disp('Weights');
  "IW{1,1}(48,:)'" : Constant  Value=[0.1675462655459337424357357804183266125619411468505859375;1.2402189577674846976407252441276796162128448486328125;0.355291129744547073965321715149912051856517791748046875;-1.086633724589072702571002082549966871738433837890625;-0.1089482361059017356819111910226638428866863250732421875;0.2946471122480260884657354836235754191875457763671875;0.56511218670757867865717116728774271905422210693359375;0.276883048011411891931032869251794181764125823974609375;-0.45315781389016984714857017024769447743892669677734375;-0.667731323895066619655835893354378640651702880859375]
      mask Display: e = 0.06;c1 = [120 150 230]/255;c2 = ([120 150 230]+0)/383;c3 = ([120 150 230]+128)/383;patch([0 1 1 0],[0 0 1 1],c1);patch([0 1 1 1-e 1-e 0+e],[0 0 1 1-e 0+e 0+e],c2);patch([0 0 1 1-e 0+e 0+e],[0 1 1 1-e 1-e 0+e],c3);plot([0 1 1 0 0],[0 0 1 1 0]);disp('Weights');
  "IW{1,1}(49,:)'" : Constant  Value=[-0.973192845927718597209832296357490122318267822265625;-0.96182970826657765428535640239715576171875;0.9680427498938339869738456400227732956409454345703125;0.27823355194579291183032410117448307573795318603515625;0.7212228374104245887110664625652134418487548828125;-0.3407914398852198711864502911339513957500457763671875;-0.71517677699934190105324205433134920895099639892578125;-0.93621861061178623941714249667711555957794189453125;0.257534866335437484519133022331516258418560028076171875;0.319853903775319914348784777757828123867511749267578125]
      mask Display: e = 0.06;c1 = [120 150 230]/255;c2 = ([120 150 230]+0)/383;c3 = ([120 150 230]+128)/383;patch([0 1 1 0],[0 0 1 1],c1);patch([0 1 1 1-e 1-e 0+e],[0 0 1 1-e 0+e 0+e],c2);patch([0 0 1 1-e 0+e 0+e],[0 1 1 1-e 1-e 0+e],c3);plot([0 1 1 0 0],[0 0 1 1 0]);disp('Weights');
  "IW{1,1}(5,:)'" : Constant  Value=[0.4395654153642085670838923761039040982723236083984375;0.30624685964174702679230222202022559940814971923828125;-0.6484890417595050582377780301612801849842071533203125;0.70454497566221785387341469686361961066722869873046875;-0.9211882977593608412547609987086616456508636474609375;0.71686970658816562274040506963501684367656707763671875;-0.37706259393198937601709985756315290927886962890625;0.12423909336177370310583256696190801449120044708251953125;-0.8453318737265289595228523467085324227809906005859375;-0.9405249105200741421839438771712593734264373779296875]
      mask Display: e = 0.06;c1 = [120 150 230]/255;c2 = ([120 150 230]+0)/383;c3 = ([120 150 230]+128)/383;patch([0 1 1 0],[0 0 1 1],c1);patch([0 1 1 1-e 1-e 0+e],[0 0 1 1-e 0+e 0+e],c2);patch([0 0 1 1-e 0+e 0+e],[0 1 1 1-e 1-e 0+e],c3);plot([0 1 1 0 0],[0 0 1 1 0]);disp('Weights');
  "IW{1,1}(50,:)'" : Constant  Value=[0.39459558799618477120674242542008869349956512451171875;0.63278840041293993312621068980661220848560333251953125;-0.607905732485043426294168966705910861492156982421875;-0.5962083261227884012356526000075973570346832275390625;0.70669960741324799879947704539517872035503387451171875;1.10941512440277190165716092451475560665130615234375;0.0678733132452306320292478858391405083239078521728515625;0.54029715712983950037795466414536349475383758544921875;1.0984466340089122926571008065366186201572418212890625;-0.0100214891146402952648575279681608662940561771392822265625]
      mask Display: e = 0.06;c1 = [120 150 230]/255;c2 = ([120 150 230]+0)/383;c3 = ([120 150 230]+128)/383;patch([0 1 1 0],[0 0 1 1],c1);patch([0 1 1 1-e 1-e 0+e],[0 0 1 1-e 0+e 0+e],c2);patch([0 0 1 1-e 0+e 0+e],[0 1 1 1-e 1-e 0+e],c3);plot([0 1 1 0 0],[0 0 1 1 0]);disp('Weights');
  "IW{1,1}(6,:)'" : Constant  Value=[0.21559703930877505140273342476575635373592376708984375;-0.62270822214827770135769924308988265693187713623046875;-0.14214929032327805469293480200576595962047576904296875;0.118766068267146973624903694144450128078460693359375;1.1853017941871362150862978523946367204189300537109375;-1.3655731685788590201724446160369552671909332275390625;0.538838735173862826144386417581699788570404052734375;-0.457585059101237534573414222904830239713191986083984375;-0.72641167223438773969945714270579628646373748779296875;-0.9793008795734305937941144293290562927722930908203125]
      mask Display: e = 0.06;c1 = [120 150 230]/255;c2 = ([120 150 230]+0)/383;c3 = ([120 150 230]+128)/383;patch([0 1 1 0],[0 0 1 1],c1);patch([0 1 1 1-e 1-e 0+e],[0 0 1 1-e 0+e 0+e],c2);patch([0 0 1 1-e 0+e 0+e],[0 1 1 1-e 1-e 0+e],c3);plot([0 1 1 0 0],[0 0 1 1 0]);disp('Weights');
  "IW{1,1}(7,:)'" : Constant  Value=[-0.11808610197136008845841814718369278125464916229248046875;-0.6908416824668106581697202273062430322170257568359375;0.724525454020324755077808731584809720516204833984375;0.7789128307291630637365642542135901749134063720703125;0.32767365722753261092492493844474665820598602294921875;0.98086444789942206501365262738545425236225128173828125;-0.313043477430321015475556123419664800167083740234375;0.57830965237321108052270801636041142046451568603515625;0.70250136040856092645157104925601743161678314208984375;-0.365783749382218636991837001914973370730876922607421875]
      mask Display: e = 0.06;c1 = [120 150 230]/255;c2 = ([120 150 230]+0)/383;c3 = ([120 150 230]+128)/383;patch([0 1 1 0],[0 0 1 1],c1);patch([0 1 1 1-e 1-e 0+e],[0 0 1 1-e 0+e 0+e],c2);patch([0 0 1 1-e 0+e 0+e],[0 1 1 1-e 1-e 0+e],c3);plot([0 1 1 0 0],[0 0 1 1 0]);disp('Weights');
  "IW{1,1}(8,:)'" : Constant  Value=[0.75706421044660887620381117812939919531345367431640625;-0.36699112977072834151925917467451654374599456787109375;-0.4104633654370613005113455074024386703968048095703125;0.98932083607724852214460042887367308139801025390625;-1.3902768089069079682218443849706090986728668212890625;0.75647677668113455506926356974872760474681854248046875;0.137138769675100469225270671813632361590862274169921875;0.7314985443610091397914629851584322750568389892578125;-0.2417898487871757706724196168579510413110256195068359375;-0.3185698308354982799528443138115108013153076171875]
      mask Display: e = 0.06;c1 = [120 150 230]/255;c2 = ([120 150 230]+0)/383;c3 = ([120 150 230]+128)/383;patch([0 1 1 0],[0 0 1 1],c1);patch([0 1 1 1-e 1-e 0+e],[0 0 1 1-e 0+e 0+e],c2);patch([0 0 1 1-e 0+e 0+e],[0 1 1 1-e 1-e 0+e],c3);plot([0 1 1 0 0],[0 0 1 1 0]);disp('Weights');
  "IW{1,1}(9,:)'" : Constant  Value=[-0.252951856736113478429928136392845772206783294677734375;-0.4698118507067208238225930472253821790218353271484375;0.8909351375051544064120889743207953870296478271484375;-0.7719319629432226381737791598425246775150299072265625;0.314759236374156647908506556632346473634243011474609375;0.54605145405481414488946256824419833719730377197265625;1.09859936731940166509957634843885898590087890625;0.455474596097248163317772196023724973201751708984375;-0.80528541514633034115178134015877731144428253173828125;-0.37130749767290838203592784338979981839656829833984375]
      mask Display: e = 0.06;c1 = [120 150 230]/255;c2 = ([120 150 230]+0)/383;c3 = ([120 150 230]+128)/383;patch([0 1 1 0],[0 0 1 1],c1);patch([0 1 1 1-e 1-e 0+e],[0 0 1 1-e 0+e 0+e],c2);patch([0 0 1 1-e 0+e 0+e],[0 1 1 1-e 1-e 0+e],c3);plot([0 1 1 0 0],[0 0 1 1 0]);disp('Weights');
  Mux : Mux  Inputs=50
      mask Display: e = 0.06;c1 = [120 150 230]/255;c2 = ([120 150 230]+0)/383;c3 = ([120 150 230]+128)/383;patch([0 1 1 0],[0 0 1 1],c1);patch([0 1 1 1-e 1-e 0+e],[0 0 1 1-e 0+e 0+e],c2);patch([0 0 1 1-e 0+e 0+e],[0 1 1 1-e 1-e 0+e],c3);plot([0 1 1 0 0],[0 0 1 1 0]);disp('Mux');
  dotprod{1..50} (50 alike) : neural/Weight Functions/dotprod
  "iz{1,1}" : Outport
      mask Display: e = 0.06;c1 = [120 230 180]/255;c2 = ([120 230 180]+0)/(256+128);c3 = ([120 230 180]+128)/(256+128);patch([0 1 1 0],[0 0 1 1],c1);patch([0 1 1 1-e 1-e 0+e],[0 0 1 1-e 0+e 0+e],c2);patch([0 0 1 1-e 0+e 0+e],[0 1 1 1-e 1-e 0+e],c3);plot([0 1 1 0 0],[0 0 1 1 0]);
  wires:
  "IW{1,1}(1,:)'"/1 -> dotprod1/1
  "pd{1,1}"/1 -> dotprod1/2, dotprod2/2, dotprod3/2, dotprod4/2, dotprod5/2, dotprod6/2, dotprod7/2, dotprod8/2, dotprod9/2, dotprod10/2, dotprod11/2, dotprod12/2, dotprod13/2, dotprod14/2, dotprod15/2, dotprod16/2, dotprod17/2, dotprod18/2, dotprod19/2, dotprod20/2, dotprod21/2, dotprod22/2, dotprod23/2, dotprod24/2, dotprod25/2, dotprod26/2, dotprod27/2, dotprod28/2, dotprod29/2, dotprod30/2, dotprod31/2, dotprod32/2, dotprod33/2, dotprod34/2, dotprod35/2, dotprod36/2, dotprod37/2, dotprod38/2, dotprod39/2, dotprod40/2, dotprod41/2, dotprod42/2, dotprod43/2, dotprod44/2, dotprod45/2, dotprod46/2, dotprod47/2, dotprod48/2, dotprod49/2, dotprod50/2
  dotprod1/1 -> Mux/1
  "IW{1,1}(2,:)'"/1 -> dotprod2/1
  dotprod2/1 -> Mux/2
  "IW{1,1}(3,:)'"/1 -> dotprod3/1
  dotprod3/1 -> Mux/3
  "IW{1,1}(4,:)'"/1 -> dotprod4/1
  dotprod4/1 -> Mux/4
  "IW{1,1}(5,:)'"/1 -> dotprod5/1
  dotprod5/1 -> Mux/5
  "IW{1,1}(6,:)'"/1 -> dotprod6/1
  dotprod6/1 -> Mux/6
  "IW{1,1}(7,:)'"/1 -> dotprod7/1
  dotprod7/1 -> Mux/7
  "IW{1,1}(8,:)'"/1 -> dotprod8/1
  dotprod8/1 -> Mux/8
  "IW{1,1}(9,:)'"/1 -> dotprod9/1
  dotprod9/1 -> Mux/9
  "IW{1,1}(10,:)'"/1 -> dotprod10/1
  dotprod10/1 -> Mux/10
  "IW{1,1}(11,:)'"/1 -> dotprod11/1
  dotprod11/1 -> Mux/11
  "IW{1,1}(12,:)'"/1 -> dotprod12/1
  dotprod12/1 -> Mux/12
  "IW{1,1}(13,:)'"/1 -> dotprod13/1
  dotprod13/1 -> Mux/13
  "IW{1,1}(14,:)'"/1 -> dotprod14/1
  dotprod14/1 -> Mux/14
  "IW{1,1}(15,:)'"/1 -> dotprod15/1
  dotprod15/1 -> Mux/15
  "IW{1,1}(16,:)'"/1 -> dotprod16/1
  dotprod16/1 -> Mux/16
  "IW{1,1}(17,:)'"/1 -> dotprod17/1
  dotprod17/1 -> Mux/17
  "IW{1,1}(18,:)'"/1 -> dotprod18/1
  dotprod18/1 -> Mux/18
  "IW{1,1}(19,:)'"/1 -> dotprod19/1
  dotprod19/1 -> Mux/19
  "IW{1,1}(20,:)'"/1 -> dotprod20/1
  dotprod20/1 -> Mux/20
  "IW{1,1}(21,:)'"/1 -> dotprod21/1
  dotprod21/1 -> Mux/21
  "IW{1,1}(22,:)'"/1 -> dotprod22/1
  dotprod22/1 -> Mux/22
  "IW{1,1}(23,:)'"/1 -> dotprod23/1
  dotprod23/1 -> Mux/23
  "IW{1,1}(24,:)'"/1 -> dotprod24/1
  dotprod24/1 -> Mux/24
  "IW{1,1}(25,:)'"/1 -> dotprod25/1
  dotprod25/1 -> Mux/25
  "IW{1,1}(26,:)'"/1 -> dotprod26/1
  dotprod26/1 -> Mux/26
  "IW{1,1}(27,:)'"/1 -> dotprod27/1
  dotprod27/1 -> Mux/27
  "IW{1,1}(28,:)'"/1 -> dotprod28/1
  dotprod28/1 -> Mux/28
  "IW{1,1}(29,:)'"/1 -> dotprod29/1
  dotprod29/1 -> Mux/29
  "IW{1,1}(30,:)'"/1 -> dotprod30/1
  dotprod30/1 -> Mux/30
  "IW{1,1}(31,:)'"/1 -> dotprod31/1
  dotprod31/1 -> Mux/31
  "IW{1,1}(32,:)'"/1 -> dotprod32/1
  dotprod32/1 -> Mux/32
  "IW{1,1}(33,:)'"/1 -> dotprod33/1
  dotprod33/1 -> Mux/33
  "IW{1,1}(34,:)'"/1 -> dotprod34/1
  dotprod34/1 -> Mux/34
  "IW{1,1}(35,:)'"/1 -> dotprod35/1
  dotprod35/1 -> Mux/35
  "IW{1,1}(36,:)'"/1 -> dotprod36/1
  dotprod36/1 -> Mux/36
  "IW{1,1}(37,:)'"/1 -> dotprod37/1
  dotprod37/1 -> Mux/37
  "IW{1,1}(38,:)'"/1 -> dotprod38/1
  dotprod38/1 -> Mux/38
  "IW{1,1}(39,:)'"/1 -> dotprod39/1
  dotprod39/1 -> Mux/39
  "IW{1,1}(40,:)'"/1 -> dotprod40/1
  dotprod40/1 -> Mux/40
  "IW{1,1}(41,:)'"/1 -> dotprod41/1
  dotprod41/1 -> Mux/41
  "IW{1,1}(42,:)'"/1 -> dotprod42/1
  dotprod42/1 -> Mux/42
  "IW{1,1}(43,:)'"/1 -> dotprod43/1
  dotprod43/1 -> Mux/43
  "IW{1,1}(44,:)'"/1 -> dotprod44/1
  dotprod44/1 -> Mux/44
  "IW{1,1}(45,:)'"/1 -> dotprod45/1
  dotprod45/1 -> Mux/45
  "IW{1,1}(46,:)'"/1 -> dotprod46/1
  dotprod46/1 -> Mux/46
  "IW{1,1}(47,:)'"/1 -> dotprod47/1
  dotprod47/1 -> Mux/47
  "IW{1,1}(48,:)'"/1 -> dotprod48/1
  dotprod48/1 -> Mux/48
  "IW{1,1}(49,:)'"/1 -> dotprod49/1
  dotprod49/1 -> Mux/49
  "IW{1,1}(50,:)'"/1 -> dotprod50/1
  dotprod50/1 -> Mux/50
  Mux/1 -> "iz{1,1}"/1
